simulink model "Caso1SemPrincipioSuperposicao"  (R2015a)
settings: Solver=ode45  StartTime=0.0  StopTime=10.0  RelTol=1e-3
settings Model: Creator=user  LastModifiedBy=user

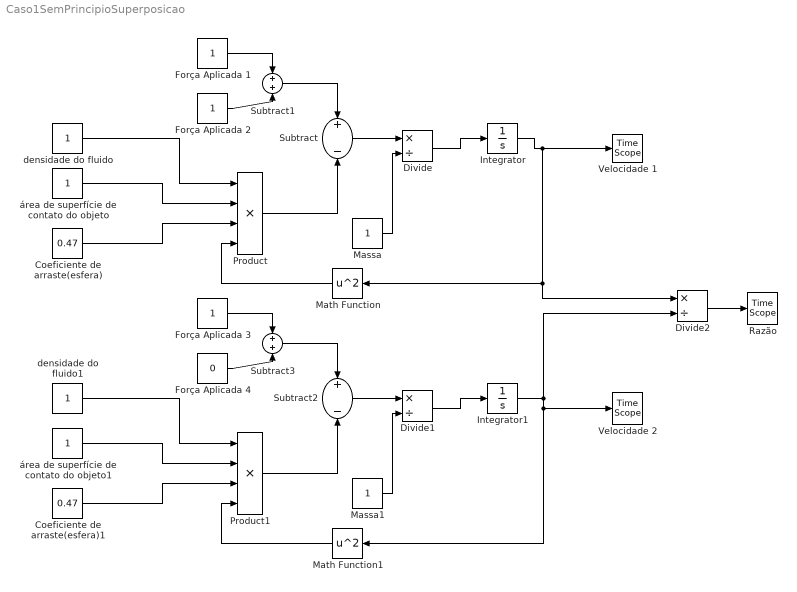
== system Caso1SemPrincipioSuperposicao ==
  Coeficiente de arraste(esfera) : Constant  Value=0.47
  Coeficiente de arraste(esfera)1 : Constant  Value=0.47
  Divide : Product  Inputs=*/
  Divide1 : Product  Inputs=*/
  Divide2 : Product  Inputs=*/
  Força Aplicada 1 : Constant
  Força Aplicada 2 : Constant
  Força Aplicada 3 : Constant
  Força Aplicada 4 : Constant  Value=0
  Integrator : Integrator
  Integrator1 : Integrator
  Massa : Constant
  Massa1 : Constant
  Math Function : Math  Operator=square  SaturateOnIntegerOverflow=on
  Math Function1 : Math  Operator=square  SaturateOnIntegerOverflow=on
  Product : Product  Inputs=4
  Product1 : Product  Inputs=4
  Razão : TimeScope
  Subtract : Sum  Inputs=+-
  Subtract1 : Sum
  Subtract2 : Sum  Inputs=+-
  Subtract3 : Sum
  Velocidade 1 : TimeScope
  Velocidade 2 : TimeScope
  densidade do fluido : Constant
  densidade do fluido1 : Constant
  área de superfície de contato do objeto : Constant
  área de superfície de contato do objeto1 : Constant
  wires:
  Product/1 -> Subtract/2
  área de superfície de contato do objeto/1 -> Product/2
  densidade do fluido/1 -> Product/1
  Coeficiente de arraste(esfera)/1 -> Product/3
  Integrator/1 -> Velocidade 1/1, Divide2/1, Math Function/1
  Math Function/1 -> Product/4
  Subtract/1 -> Divide/1
  Divide/1 -> Integrator/1
  Massa/1 -> Divide/2
  Força Aplicada 1/1 -> Subtract1/1
  Força Aplicada 2/1 -> Subtract1/2
  Subtract1/1 -> Subtract/1
  Product1/1 -> Subtract2/2
  área de superfície de contato do objeto1/1 -> Product1/2
  densidade do fluido1/1 -> Product1/1
  Coeficiente de arraste(esfera)1/1 -> Product1/3
  Integrator1/1 -> Math Function1/1, Velocidade 2/1, Divide2/2
  Math Function1/1 -> Product1/4
  Subtract2/1 -> Divide1/1
  Divide1/1 -> Integrator1/1
  Massa1/1 -> Divide1/2
  Força Aplicada 3/1 -> Subtract3/1
  Força Aplicada 4/1 -> Subtract3/2
  Subtract3/1 -> Subtract2/1
  Divide2/1 -> Razão/1
